simulink model "motor_model_sim"  (R2022a)
settings: Solver=ode23t  StartTime=0.0  StopTime=7  FixedStep=0.001  RelTol=1e-3
values from neighbouring files (symbols this model uses):
  A = [-0.236727989131  0  223.542179776; -420.783816284  -0.236727989131  -1280.33188497; -1.88234639523  0  -5.72747338445]    [mechanics_explorer.mat]
  B = [115.011055472  0; 0  216.959927767; 0  0.970554765031]    [mechanics_explorer.mat]
  C = [1  0  0; 0  1  0; 0  0  1]    [mechanics_explorer.mat]
  D = [0 0 0]    [mechanics_explorer.mat]
  Km = 1.94365818885    [mechanics_explorer.mat]
undefined symbols (not defined in the file or in its folder): Const_input, U_nominal
libraries: slpidlib x1
settings Model: Creator=asmax  LastModifiedBy=Maxim
settings SolverCC: EnableFixedStepZeroCrossing=on

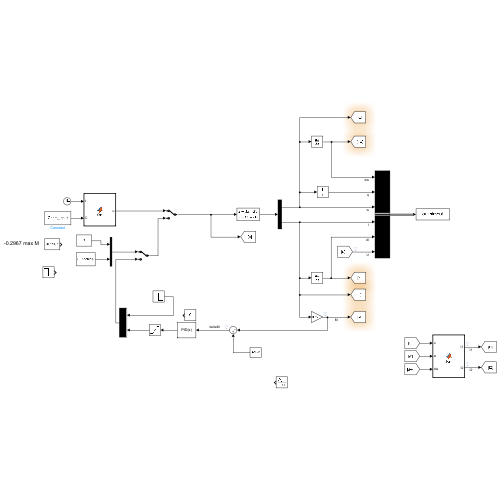
[thumbnail: Simulink's stored preview of the top-level diagram]
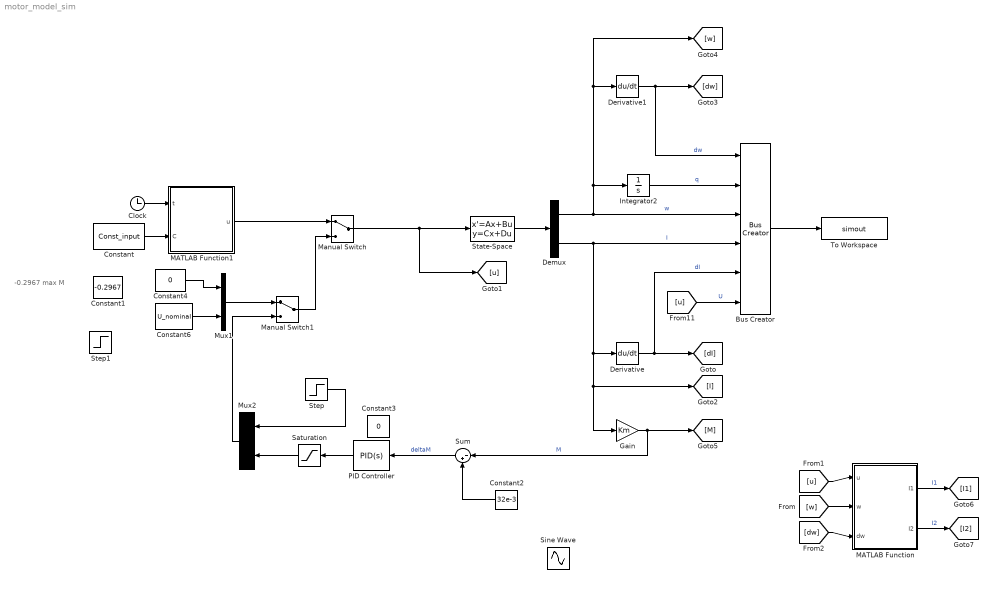
== system motor_model_sim ==
  note: -0.2967 max M
  Bus Creator : BusCreator  Inputs=6
  Clock : Clock
  Constant : Constant  Value=Const_input
  Constant1 : Constant  Value=-0.2967
  Constant2 : Constant  Value=32e-3
  Constant3 : Constant  Value=0
  Constant4 : Constant  Value=0
  Constant6 : Constant  Value=U_nominal
  Demux : Demux  Outputs=2
  Derivative : Derivative
  Derivative1 : Derivative
  Gain : Gain  Gain=Km
  Integrator2 : Integrator
  MATLAB Function : MATLAB Function  TreatAsAtomicUnit=on
  MATLAB Function1 : MATLAB Function  TreatAsAtomicUnit=on
  Manual Switch : ManualSwitch
  Manual Switch1 : ManualSwitch
  Mux1 : Mux  Inputs=2
  Mux2 : Mux  Inputs=2
  PID Controller : slpidlib/PID Controller  Controller=PID  Form=Parallel  TimeDomain=Continuous-time  UseExternalTs=off  SampleTime=-1  IntegratorMethod=Forward Euler  FilterMethod=Forward Euler  ControllerParametersSource=internal  P=1e4  I=1  UseKiTs=off  D=1e2  N=100  UseFilter=on  TunerSelectOption=Transfer Function Based (PID Tuner App)  InitialConditionSource=internal  InitialConditionForIntegrator=0  InitialConditionForFilter=0  DifferentiatorICPrevScaledInput=0  ExternalReset=none  TrackingMode=off  Kt=1  LimitOutput=off  SatLimitsSource=internal  UpperSaturationLimit=inf  LowerSaturationLimit=-inf  LinearizeAsGain=on  AntiWindupMode=none  Kb=1  POutMin=[]  POutMax=[]  IOutMin=[]  IOutMax=[]  DOutMin=[]  DOutMax=[]  NOutMin=[]  NOutMax=[]  SumOutMin=[]  SumOutMax=[]  SaturationOutMin=[]  SaturationOutMax=[]  PParamMin=[]  PParamMax=[]  IParamMin=[]  IParamMax=[]  DParamMin=[]  DParamMax=[]  NParamMin=[]  NParamMax=[]  KbParamMin=[]  KbParamMax=[]  KtParamMin=[]  KtParamMax=[]  KbOutMin=[]  KbOutMax=[]  KtOutMin=[]  KtOutMax=[]  IntegratorOutMin=[]  IntegratorOutMax=[]  FilterOutMin=[]  FilterOutMax=[]  SumI1OutMin=[]  SumI1OutMax=[]  SumI2OutMin=[]  SumI2OutMax=[]  SumI3OutMin=[]  SumI3OutMax=[]  SumI4OutMin=[]  SumI4OutMax=[]  SumDOutMin=[]  SumDOutMax=[]  DifferentiatorOutMin=[]  DifferentiatorOutMax=[]  FilterDiffOutCoefMin=[]  FilterDiffOutCoefMax=[]  ReciprocalOutMin=[]  ReciprocalOutMax=[]  SumDenOutMin=[]  SumDenOutMax=[]  SumNumOutMin=[]  SumNumOutMax=[]  DivideOutMin=[]  DivideOutMax=[]  UdiffTsProdOutMin=[]  UdiffTsProdOutMax=[]  NTsProdOutMin=[]  NTsProdOutMax=[]  UintegralTsProdOutMin=[]  UintegralTsProdOutMax=[]  UngainTsProdOutMin=[]  UngainTsProdOutMax=[]  IntegratorContinuousStateAttributes=''  IntegratorStateMustResolveToSignalObject=off  IntegratorRTWStateStorageClass=Auto  FilterContinuousStateAttributes=''  FilterStateMustResolveToSignalObject=off  FilterRTWStateStorageClass=Auto  ParallelPVariant=InternalParameters  IdealPVariant=Disabled  IVariant=InternalParameters  DVariant=InternalParameters  IntegratorVariant=Continuous  SatVariant=Disabled  AWVariant=Passthrough  PCopyVariant=Disabled  TRVariant=Disabled  FdbkBlocksVariant=Forward  IdealPFdbkVariant=Disabled  SatFdbkVariant=Disabled  DerivativeFilterVariant=ContFilter  NVariant=InternalParameters  NCopyVariant=Disabled  FilterICVariant=InternalICsFilter  IntegratorICVariant=InternalICs  ExternalResetVariant=Disabled  TRSumVariant=Passthrough  SumFdbkVariant=Disabled  SumVariant=Sum_PID  TsampFilterVariant=InternalTs  TsampNgainVariant=Passthrough  TsampIntegralVariant=Passthrough  ExternalSaturationOutDataTypeStr=Inherit: Same as second input  aMode=0
  Saturation : Saturate  UpperLimit=U_nominal  LowerLimit=-U_nominal
  Sine Wave : Sin  Amplitude=32e-3  SampleTime=0
  State-Space : StateSpace  A=A  B=B  C=C  D=D  InitialCondition=[0;0]
  Step : Step  Time=4  After=-32e-3  SampleTime=0
  Step1 : Step  Time=4  After=-32e-3  SampleTime=0
  Sum : Sum  Inputs=|-+
  To Workspace : ToWorkspace  VariableName=simout  SaveFormat=Timeseries  SampleTime=-1
  wires:
  Manual Switch/1 -> State-Space/1, [u]
  State-Space/1 -> Demux/1
  Demux/1 -> Integrator2/1, [w], Derivative1/1, Bus Creator/3  "w"
  Demux/2 -> Bus Creator/4, Gain/1, [I], Derivative/1  "I"
  Bus Creator/1 -> To Workspace/1
  Derivative/1 -> Bus Creator/5, [dI]  "dI"
  Derivative1/1 -> [dw], Bus Creator/1  "dw"
  Clock/1 -> MATLAB Function1/1(t)
  MATLAB Function1/1(u) -> Manual Switch/1
  Integrator2/1 -> Bus Creator/2  "q"
  [u] -> Bus Creator/6  "U"
  Constant/1 -> MATLAB Function1/2(C)
  Constant6/1 -> Mux1/2
  Gain/1 -> Sum/1, [M]  "M"
  Mux1/1 -> Manual Switch1/1
  Manual Switch1/1 -> Manual Switch/2
  Sum/1 -> PID Controller/1  "deltaM"
  Mux2/1 -> Manual Switch1/2
  PID Controller/1 -> Saturation/1
  Saturation/1 -> Mux2/2
  Step/1 -> Mux2/1
  Constant2/1 -> Sum/2
  [u] -> MATLAB Function/1(u)
  [w] -> MATLAB Function/2(w)
  [dw] -> MATLAB Function/3(dw)
  MATLAB Function/1(I1) -> [I1]  "I1"
  MATLAB Function/2(I2) -> [I2]  "I2"
  Constant4/1 -> Mux1/1

== matlab function motor_model_sim/MATLAB Function ==
  data: u input; I1 output; w input; dw input; I2 output
function [I1, I2] = fcn(u, w, dw)

Km = 0.2923;
Kw = -0.2923;
Lam = 0.0019*1.53 ;
J = 0.0011*2;
R = 11.8227*16;

Km = 0.2923;
Kw = 0.2923;
Lam = 0.0019;
J = 0.0011;
R = 11.8227;

input = u(2);

I1 = J*dw + Lam*w;
I2 = (input - Kw*w)/R;

== matlab function motor_model_sim/MATLAB Function1 ==
  data: t input; u output; C input
function u = fcn(t, C)

w = C(3);
A = C(1);
B = C(2);
fi = C(4);
u = [C(5) A * cos(w * t*2*pi + fi) + B]';
